simulink model "Q1sim"  (R2023a)
settings: Solver=FixedStepAuto  StartTime=0.0  StopTime=simulation_end_time  FixedStep=integration_step_time  RelTol=1e-3
values from neighbouring files (symbols this model uses):
  b = 0.009    [main.m]
  J = 0.0051    [main.m]
  K_b = 0.024    [main.m]
  K_m = 24e-3    (= 0.024)    [main.m]
  K_u = 1.2    [main.m]
  L_a = 0    [main.m]
  N_r = 57/11    (= 5.18181818182)    [main.m]
  R_a = 2.08    [main.m]
  simulation_start_time = 0    [main.m]
  T_d = 0    [main.m]
  u_t = 1    [main.m]
settings Model: Creator=אלמוג  LastModifiedBy=אלמוג

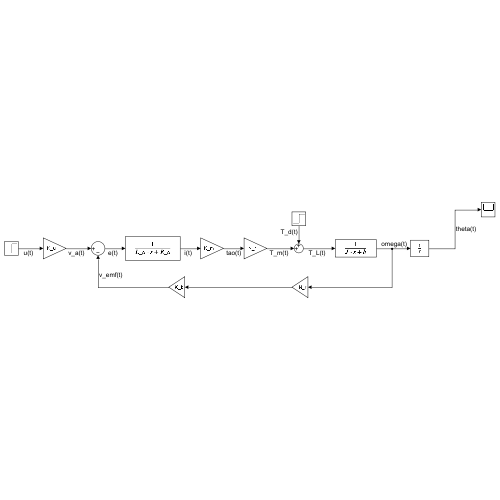
[thumbnail: Simulink's stored preview of the top-level diagram]
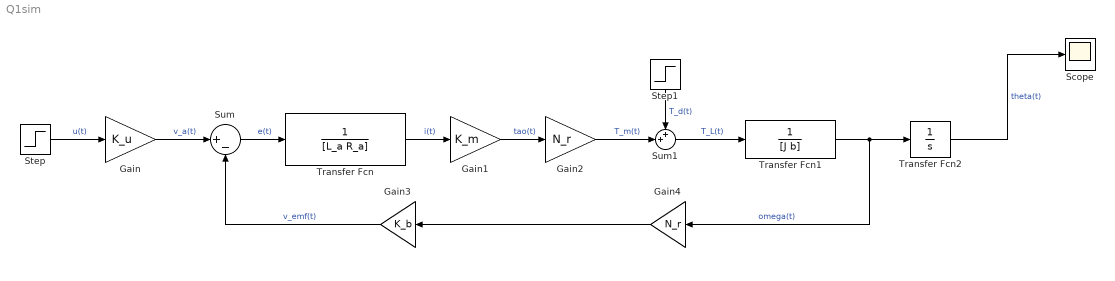
== system Q1sim ==
  Gain : Gain  Gain=K_u
  Gain1 : Gain  Gain=K_m
  Gain2 : Gain  Gain=N_r
  Gain3 : Gain  Gain=K_b
  Gain4 : Gain  Gain=N_r
  Scope : Scope
  Step : Step  Time=simulation_start_time  After=u_t  SampleTime=0
  Step1 : Step  Time=simulation_start_time  After=T_d  SampleTime=0
  Sum : Sum  Inputs=|+-
  Sum1 : Sum  Inputs=++|
  Transfer Fcn : TransferFcn  Denominator=[L_a R_a]
  Transfer Fcn1 : TransferFcn  Denominator=[J b]
  Transfer Fcn2 : TransferFcn  Denominator=[1 0]
  wires:
  Step/1 -> Gain/1  "u(t)"
  Gain/1 -> Sum/1  "v_a(t)"
  Sum/1 -> Transfer Fcn/1  "e(t)"
  Transfer Fcn/1 -> Gain1/1  "i(t)"
  Gain1/1 -> Gain2/1  "tao(t)"
  Gain2/1 -> Sum1/2  "T_m(t)"
  Step1/1 -> Sum1/1  "T_d(t)"
  Sum1/1 -> Transfer Fcn1/1  "T_L(t)"
  Transfer Fcn1/1 -> Gain4/1, Transfer Fcn2/1  "omega(t)"
  Transfer Fcn2/1 -> Scope/1  "theta(t)"
  Gain3/1 -> Sum/2  "v_emf(t)"
  Gain4/1 -> Gain3/1
